simulink model "ctof"  (R2013a)
settings: Solver=ode45  StartTime=0.0  StopTime=10.0  RelTol=1e-3
settings Model: Creator=teslian  LastModifiedBy=teslian

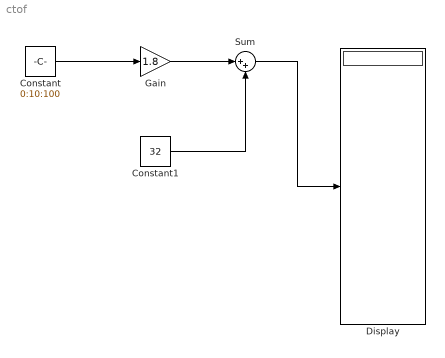
== system ctof ==
  Constant : Constant  Value=0:10:100
  Constant1 : Constant  Value=32
  Display : Display
  Gain : Gain  Gain=1.8
  Sum : Sum  Inputs=|++
  wires:
  Sum/1 -> Display/1
  Constant1/1 -> Sum/2
  Gain/1 -> Sum/1
  Constant/1 -> Gain/1
